simulink model "Motor CC"  (R2017a)
settings: Solver=VariableStepAuto  StartTime=0.0  StopTime=2.0  RelTol=1e-3
undefined symbols (not defined in the file): B, J, kb, km, La, Ra
settings Model: Creator=vbobarth  LastModifiedBy=vbobarth

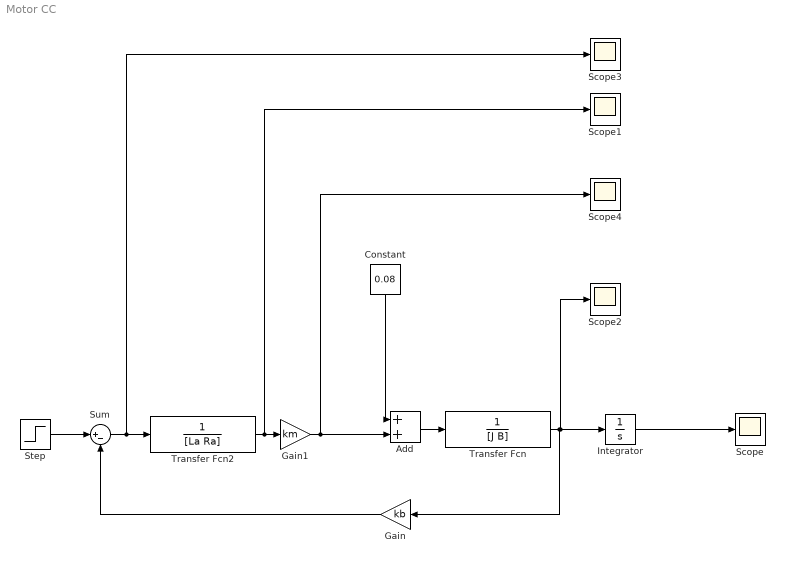
== system Motor CC ==
  Add : Sum
  Constant : Constant  Value=0.08
  Gain : Gain  Gain=kb
  Gain1 : Gain  Gain=km
  Integrator : Integrator
  Scope{,1..4} (5 alike) : Scope
  Step : Step  SampleTime=0
  Sum : Sum  Inputs=|+-
  Transfer Fcn : TransferFcn  Denominator=[J B]
  Transfer Fcn2 : TransferFcn  Denominator=[La Ra]
  wires:
  Transfer Fcn/1 -> Scope2/1, Integrator/1, Gain/1
  Gain/1 -> Sum/2
  Add/1 -> Transfer Fcn/1
  Gain1/1 -> Scope4/1, Add/2
  Constant/1 -> Add/1
  Integrator/1 -> Scope/1
  Sum/1 -> Transfer Fcn2/1, Scope3/1
  Transfer Fcn2/1 -> Scope1/1, Gain1/1
  Step/1 -> Sum/1
